simulink model "EtherNet_test"  (R2025a)
settings: Solver=VariableStepAuto  StartTime=0.0  StopTime=inf  RelTol=1e-3
libraries: slrealtimeiplib x2, sldrtlib x1
settings Model: Creator=xuejf  LastModifiedBy=xuejf

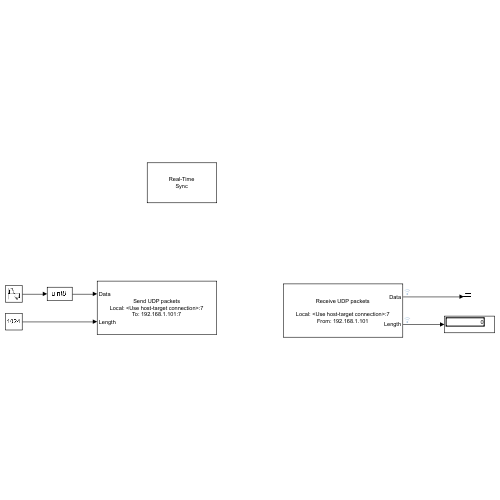
[thumbnail: Simulink's stored preview of the top-level diagram]
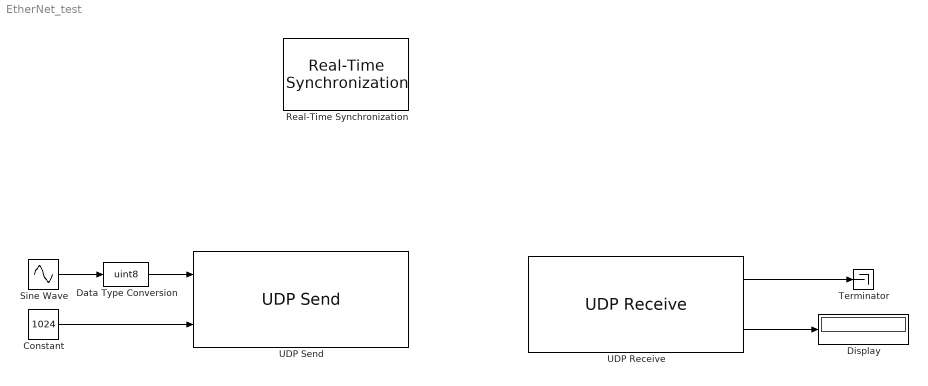
== system EtherNet_test ==
  Constant : Constant  Value=1024
  Data Type Conversion : DataTypeConversion  OutDataTypeStr=uint8  SaturateOnIntegerOverflow=off  RndMeth=Floor
  Display : Display
  Real-Time Synchronization : sldrtlib/Real-Time Synchronization  SampleTime=0.0001  MaxMissedTicks=1000  ShowMissedTicks=off  YieldWhenWaiting=off
  Sine Wave : Sin  Amplitude=64  Bias=128  Frequency=2*pi  Phase=linspace(0,2*pi,1024)  SampleTime=1e-3
  Terminator : Terminator
  UDP Receive : slrealtimeiplib/UDP Receive  useHostTargetConn=on  ipAddress=10.10.10.15  localPort=7  rcvWidth=1024  rcvFmAny=off  fmAddress=192.168.1.101  sampleTime=0.001  enableMessage=off  maxPackets=1
  UDP Send : slrealtimeiplib/UDP Send  useHostTargetConn=on  toAddress=192.168.1.101  toPort=7  sampleTime=0.001  enableMessage=off  localPort=7
  wires:
  Sine Wave/1 -> Data Type Conversion/1
  Data Type Conversion/1 -> UDP Send/1
  Constant/1 -> UDP Send/2
  UDP Receive/2 -> Display/1
  UDP Receive/1 -> Terminator/1
